simulink model "Traffic_Light_ROS2_NS3_demo"  (R2024b)
settings: Solver=ode3  StartTime=0.0  StopTime=100  FixedStep=0.001  MaxStep=0.05  RelTol=1e-3
model workspace (MAT data in the model file):
  SL_ROS_VariableLengthArrays_MaxSizes.CommonInfo.ArrayTruncateAction = 'EmitWarning'
  SL_ROS_VariableLengthArrays_MaxSizes.MsgTypeMap = containers.Map
  SL_ROS_VariableLengthArrays_MaxSizes.MsgTypeMap.serialization.keys = {'nav_msgs/Path', 'sensor_msgs/Image', 'sensor_msgs/PointCloud2'}
  SL_ROS_VariableLengthArrays_MaxSizes.MsgTypeMap.serialization.values{1}.PropertyName = 'poses'
  SL_ROS_VariableLengthArrays_MaxSizes.MsgTypeMap.serialization.values{1}.DataType = 'geometry_msgs/PoseStamped'
  SL_ROS_VariableLengthArrays_MaxSizes.MsgTypeMap.serialization.values{1}.MaxLength = 1000
  SL_ROS_VariableLengthArrays_MaxSizes.MsgTypeMap.serialization.values{2}(1).PropertyName = 'data'
  SL_ROS_VariableLengthArrays_MaxSizes.MsgTypeMap.serialization.values{2}(1).DataType = 'uint8'
  SL_ROS_VariableLengthArrays_MaxSizes.MsgTypeMap.serialization.values{2}(1).MaxLength = 2000000
  SL_ROS_VariableLengthArrays_MaxSizes.MsgTypeMap.serialization.values{2}(2).PropertyName = 'encoding'
  SL_ROS_VariableLengthArrays_MaxSizes.MsgTypeMap.serialization.values{2}(2).DataType = 'uint8'
  SL_ROS_VariableLengthArrays_MaxSizes.MsgTypeMap.serialization.values{2}(2).MaxLength = 2000000
  SL_ROS_VariableLengthArrays_MaxSizes.MsgTypeMap.serialization.values{3}(1).PropertyName = 'data'
  SL_ROS_VariableLengthArrays_MaxSizes.MsgTypeMap.serialization.values{3}(1).DataType = 'uint8'
  SL_ROS_VariableLengthArrays_MaxSizes.MsgTypeMap.serialization.values{3}(1).MaxLength = 1000000
  SL_ROS_VariableLengthArrays_MaxSizes.MsgTypeMap.serialization.values{3}(2).PropertyName = 'fields'
  SL_ROS_VariableLengthArrays_MaxSizes.MsgTypeMap.serialization.values{3}(2).DataType = 'sensor_msgs/PointField'
  SL_ROS_VariableLengthArrays_MaxSizes.MsgTypeMap.serialization.values{3}(2).MaxLength = 16
  SL_ROS_VariableLengthArrays_MaxSizes.MsgTypeMap.serialization.uniformity = 0
  SL_ROS_VariableLengthArrays_MaxSizes.MsgTypeMap.serialization.keyType = 'char'
  SL_ROS_VariableLengthArrays_MaxSizes.MsgTypeMap.serialization.valueType = 'any'
undefined symbols (not defined in the file or in its folder): brake, gear, hand_brake, manual_gear_shift, reverse, steer, throttle
libraries: ros2lib x5, slpidlib x1, instrumentlib x1
settings Model: PacingRate=0.010000  Creator=iotav  LastModifiedBy=hnh21
settings OptimizationCC: DefaultParameterBehavior=Inlined  EnhancedBackFolding=on  PassReuseOutputArgsAs=Individual arguments  ZeroExternalMemoryAtStartup=off  ZeroInternalMemoryAtStartup=off  MaxStackSize=64  OptimizeBlockOrder=speed  DifferentSizesBufferReuse=on  EfficientTunableParamExpr=on
settings DebuggingCC: ParameterTunabilityLossMsg=error
settings HardwareCC: ProdBitPerLong=64  ProdHWDeviceType=Intel->x86-64 (Linux 64)
settings RTWCC: Description=Embedded Coder  SystemTargetFile=ert.tlc  HardwareBoard=Robot Operating System 2 (ROS 2)  TLCOptions="-aInlineSetEventsForThisBaseRateFcn=TLC_FALSE -aSuppressMultiTaskScheduler=TLC_FALSE  -aRateBasedStepFcn=0"  TemplateMakefile=ert_default_tmf  Toolchain=Colcon Tools  TargetLang=C++
settings CodeAppCC: ForceParamTrailComments=on  IgnoreCustomStorageClasses=off  OperatorAnnotations=on  SimulinkDataObjDesc=on  SFDataObjDesc=on  InsertBlockDesc=on
settings ERTTargetCC: CodeInterfacePackaging=C++ class  RootIOFormat=Structure reference

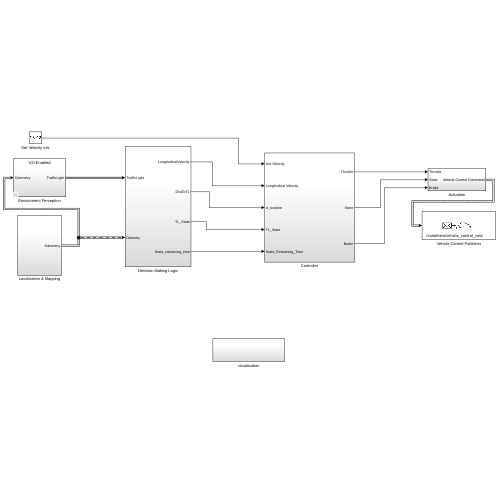
[thumbnail: Simulink's stored preview of the top-level diagram]
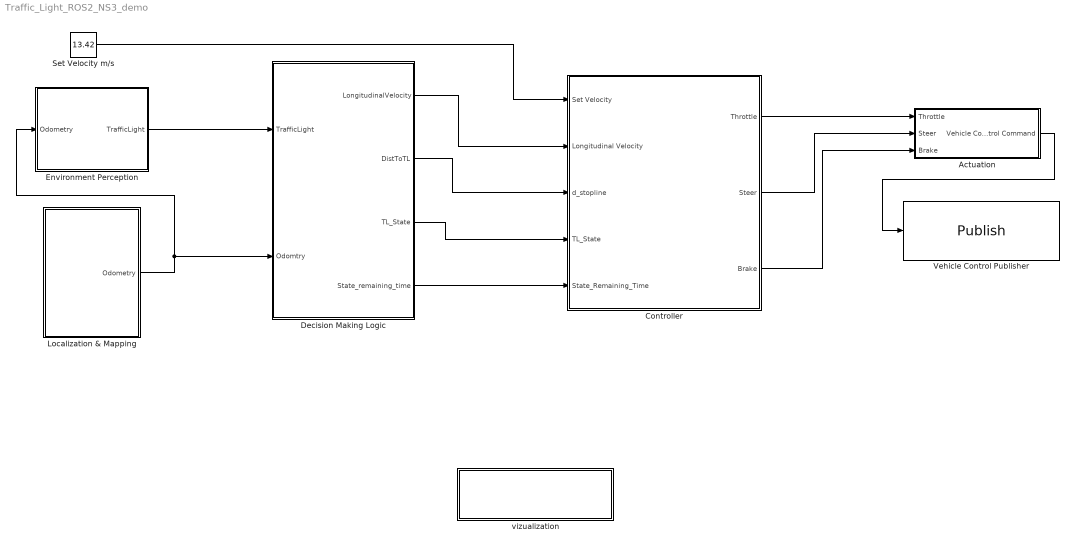
== system Traffic_Light_ROS2_NS3_demo ==
  Actuation : Subsystem
  Controller : Subsystem
  Decision Making Logic : Subsystem
  Environment Perception : Subsystem  Variant=on
  Localization & Mapping : Subsystem
  Set Velocity m/s : Constant  Value=13.42
  Vehicle Control Publisher : ros2lib/Publish  topicSource=Select from ROS network  topic=/carla/hero/vehicle_control_cmd  messageType=carla_msgs/CarlaEgoVehicleControl  QOSHistory=Keep last  QOSDepth=1  QOSReliability=Reliable  QOSDurability=Volatile  QOSDeadline=Inf  QOSLifespan=Inf  QOSLiveliness=Automatic  QOSLeaseDuration=Inf  QOSAvoidROSNamespaceConventions=off
  vizualization : Subsystem
  wires:
  Environment Perception/1(TrafficLight) -> Decision Making Logic/1(TrafficLight)
  Localization & Mapping/1(Odometry) -> Environment Perception/1(Odometry), Decision Making Logic/2(Odomtry)
  Actuation/1(Vehicle Control Command) -> Vehicle Control Publisher/1
  Set Velocity m/s/1 -> Controller/1(Set Velocity)
  Decision Making Logic/1(LongitudinalVelocity) -> Controller/2(Longitudinal Velocity)
  Decision Making Logic/2(DistToTL) -> Controller/3(d_stopline)
  Decision Making Logic/3(TL_State) -> Controller/4(TL_State)
  Controller/1(Throttle) -> Actuation/1(Throttle)
  Controller/2(Steer) -> Actuation/2(Steer)
  Controller/3(Brake) -> Actuation/3(Brake)
  Decision Making Logic/4(State_remaining_time) -> Controller/5(State_Remaining_Time)

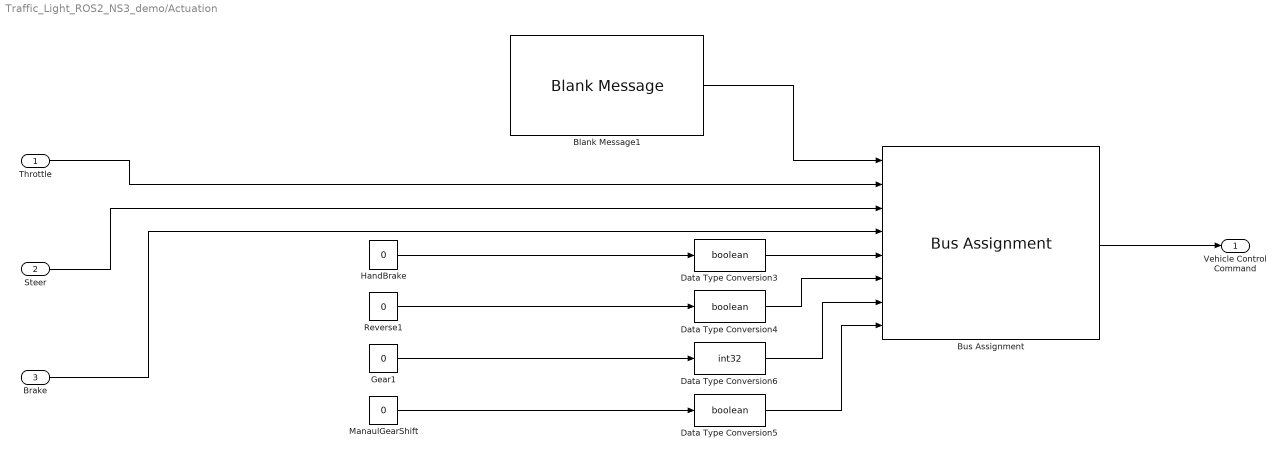
== system Traffic_Light_ROS2_NS3_demo/Actuation ==
  Throttle : Inport
  Steer : Inport  Port=2
  Brake : Inport  Port=3
  Blank Message1 : ros2lib/Blank Message  messageClass=Message  entityType=carla_msgs/CarlaEgoVehicleControl  messageType=carla_msgs/CarlaEgoVehicleControl  SampleTime=inf
  Bus Assignment : BusAssignment  AssignedSignals=throttle,steer,brake,hand_brake,reverse,gear,manual_gear_shift
  Data Type Conversion3 : DataTypeConversion  OutDataTypeStr=boolean  SaturateOnIntegerOverflow=off  RndMeth=Floor
  Data Type Conversion4 : DataTypeConversion  OutDataTypeStr=boolean  SaturateOnIntegerOverflow=off  RndMeth=Floor
  Data Type Conversion5 : DataTypeConversion  OutDataTypeStr=boolean  SaturateOnIntegerOverflow=off  RndMeth=Floor
  Data Type Conversion6 : DataTypeConversion  OutDataTypeStr=int32  SaturateOnIntegerOverflow=off  RndMeth=Floor
  Gear1 : Constant  Value=0  OutDataTypeStr=single
  HandBrake : Constant  Value=0  OutDataTypeStr=single
  ManaulGearShift : Constant  Value=0  OutDataTypeStr=single
  Reverse1 : Constant  Value=0  OutDataTypeStr=single
  Vehicle Control Command : Outport
  wires:
  Data Type Conversion5/1 -> Bus Assignment/8
  Data Type Conversion6/1 -> Bus Assignment/7
  Blank Message1/1 -> Bus Assignment/1
  Data Type Conversion4/1 -> Bus Assignment/6
  Data Type Conversion3/1 -> Bus Assignment/5
  Throttle/1 -> Bus Assignment/2
  Bus Assignment/1 -> Vehicle Control Command/1
  Steer/1 -> Bus Assignment/3
  Brake/1 -> Bus Assignment/4
  HandBrake/1 -> Data Type Conversion3/1
  Reverse1/1 -> Data Type Conversion4/1
  Gear1/1 -> Data Type Conversion6/1
  ManaulGearShift/1 -> Data Type Conversion5/1

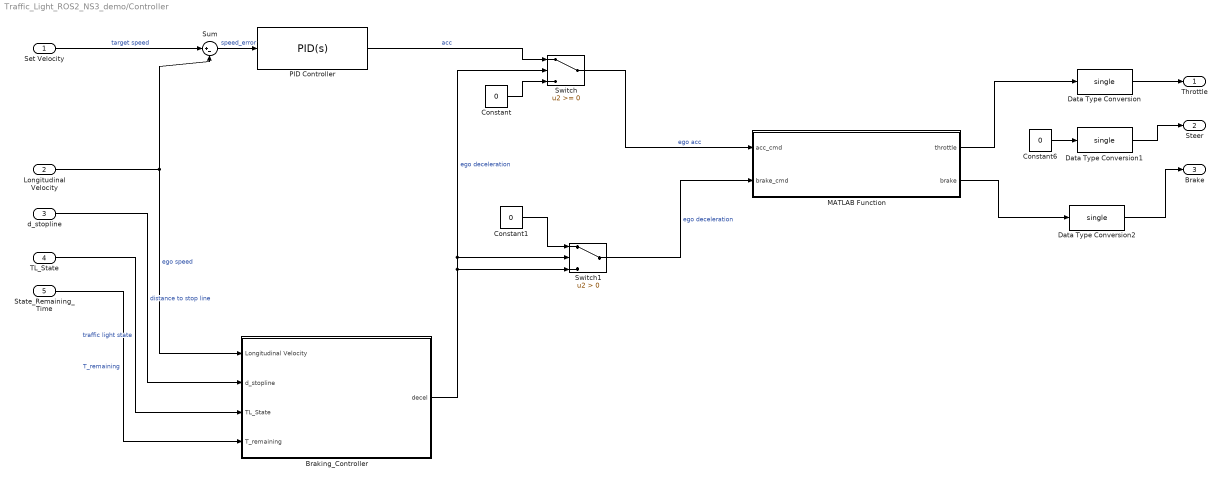
== system Traffic_Light_ROS2_NS3_demo/Controller ==
  Set Velocity : Inport
  Longitudinal Velocity : Inport  Port=2
  d_stopline : Inport  Port=3
  TL_State : Inport  Port=4
  State_Remaining_Time : Inport  Port=5
  Braking_Controller : Subsystem  Variant=on  VariantControl=BRAKING_MODE
  Constant : Constant  Value=0
  Constant1 : Constant  Value=0
  Constant6 : Constant  Value=0
  Data Type Conversion : DataTypeConversion  OutDataTypeStr=single  SaturateOnIntegerOverflow=off  RndMeth=Floor
  Data Type Conversion1 : DataTypeConversion  OutDataTypeStr=single  SaturateOnIntegerOverflow=off  RndMeth=Floor
  Data Type Conversion2 : DataTypeConversion  OutDataTypeStr=single  SaturateOnIntegerOverflow=off  RndMeth=Floor
  MATLAB Function : MATLAB Function  TreatAsAtomicUnit=on
  PID Controller : slpidlib/PID Controller  Controller=PID  Form=Parallel  TimeDomain=Continuous-time  UseExternalTs=off  SampleTime=-1  IntegratorMethod=Forward Euler  FilterMethod=Forward Euler  ControllerParametersSource=internal  P=0.6  I=0.1  UseKiTs=off  D=0  UseExternalDerivativeSource=off  N=100  UseFilter=on  TunerSelectOption=Transfer Function Based (PID Tuner App)  InitialConditionSource=internal  InitialConditionForIntegrator=0  InitialConditionForFilter=0  DifferentiatorICPrevScaledInput=0  ExternalReset=none  TrackingMode=off  Kt=1  LimitOutput=on  SatLimitsSource=internal  UpperSaturationLimit=2  LowerSaturationLimit=-3  LinearizeAsGain=on  AntiWindupMode=none  Kb=1  LimitIntegrator=off  UpperIntegratorSaturationLimit=inf  LowerIntegratorSaturationLimit=-inf  POutMin=[]  POutMax=[]  IOutMin=[]  IOutMax=[]  DOutMin=[]  DOutMax=[]  NOutMin=[]  NOutMax=[]  SumOutMin=[]  SumOutMax=[]  SaturationOutMin=[]  SaturationOutMax=[]  PParamMin=[]  PParamMax=[]  IParamMin=[]  IParamMax=[]  DParamMin=[]  DParamMax=[]  NParamMin=[]  NParamMax=[]  KbParamMin=[]  KbParamMax=[]  KtParamMin=[]  KtParamMax=[]  KbOutMin=[]  KbOutMax=[]  KtOutMin=[]  KtOutMax=[]  IntegratorOutMin=[]  IntegratorOutMax=[]  FilterOutMin=[]  FilterOutMax=[]  SumI1OutMin=[]  SumI1OutMax=[]  SumI2OutMin=[]  SumI2OutMax=[]  SumI3OutMin=[]  SumI3OutMax=[]  SumI4OutMin=[]  SumI4OutMax=[]  SumDOutMin=[]  SumDOutMax=[]  DifferentiatorOutMin=[]  DifferentiatorOutMax=[]  FilterDiffOutCoefMin=[]  FilterDiffOutCoefMax=[]  ReciprocalOutMin=[]  ReciprocalOutMax=[]  SumDenOutMin=[]  SumDenOutMax=[]  SumNumOutMin=[]  SumNumOutMax=[]  DivideOutMin=[]  DivideOutMax=[]  UdiffTsProdOutMin=[]  UdiffTsProdOutMax=[]  NTsProdOutMin=[]  NTsProdOutMax=[]  UintegralTsProdOutMin=[]  UintegralTsProdOutMax=[]  UngainTsProdOutMin=[]  UngainTsProdOutMax=[]  ClampingZeroOutDataTypeStr=Inherit: Inherit via back propagation  ClampingZeroOutMin=[]  ClampingZeroOutMax=[]  FilterDenConstantOutDataTypeStr=Inherit: Inherit via back propagation  FilterDenConstantOutMin=[]  FilterDenConstantOutMax=[]  PCopyOutDataTypeStr=Inherit: Inherit via back propagation  PCopyOutMin=[]  PCopyOutMax=[]  NCopyOutDataTypeStr=Inherit: Inherit via back propagation  NCopyOutMin=[]  NCopyOutMax=[]  IntegratorContinuousStateAttributes=''  IntegratorStateMustResolveToSignalObject=off  IntegratorRTWStateStorageClass=Auto  FilterContinuousStateAttributes=''  FilterStateMustResolveToSignalObject=off  FilterRTWStateStorageClass=Auto  ParallelPVariant=InternalParameters  IdealPVariant=Disabled  IVariant=InternalParameters  DVariant=InternalParameters  IntegratorVariant=Continuous  SatVariant=Enabled  AWVariant=Passthrough  PCopyVariant=Disabled  TRVariant=Disabled  FdbkBlocksVariant=Forward  IdealPFdbkVariant=Disabled  SatFdbkVariant=Disabled  DerivativeFilterVariant=ContFilter  NVariant=InternalParameters  NCopyVariant=Disabled  FilterICVariant=InternalICsFilter  IntegratorICVariant=InternalICs  ExternalResetVariant=Disabled  TRSumVariant=Passthrough  SumFdbkVariant=Disabled  SumVariant=Sum_PID  TsampFilterVariant=InternalTs  TsampNgainVariant=Passthrough  TsampIntegralVariant=Disabled_SignalSpec  ExternalSaturationOutDataTypeStr=Inherit: Same as second input  DerivativeSourceVariant=ErrorSignal  PreIntVariant=InternalPreInt
  Sum : Sum  Inputs=|+-
  Switch : Switch  SaturateOnIntegerOverflow=off  InputSameDT=off
  Switch1 : Switch  Criteria=u2 > Threshold  SaturateOnIntegerOverflow=off  InputSameDT=off
  Throttle : Outport
  Steer : Outport  Port=2
  Brake : Outport  Port=3
  wires:
  Constant6/1 -> Data Type Conversion1/1
  d_stopline/1 -> Braking_Controller/2(d_stopline)  "distance to stop line"
  MATLAB Function/1(throttle) -> Data Type Conversion/1
  Set Velocity/1 -> Sum/1  "target speed"
  Data Type Conversion2/1 -> Brake/1
  Sum/1 -> PID Controller/1  "speed_error"
  TL_State/1 -> Braking_Controller/3(TL_State)  "traffic light state"
  MATLAB Function/2(brake) -> Data Type Conversion2/1
  Data Type Conversion/1 -> Throttle/1
  Braking_Controller/1(decel) -> Switch1/3, Switch/2, Switch1/2  "ego deceleration"
  Data Type Conversion1/1 -> Steer/1
  Longitudinal Velocity/1 -> Braking_Controller/1(Longitudinal Velocity), Sum/2  "ego speed"
  PID Controller/1 -> Switch/1  "acc"
  Switch/1 -> MATLAB Function/1(acc_cmd)  "ego acc"
  Constant/1 -> Switch/3
  State_Remaining_Time/1 -> Braking_Controller/4(T_remaining)  "T_remaining"
  Switch1/1 -> MATLAB Function/2(brake_cmd)  "ego deceleration"
  Constant1/1 -> Switch1/1

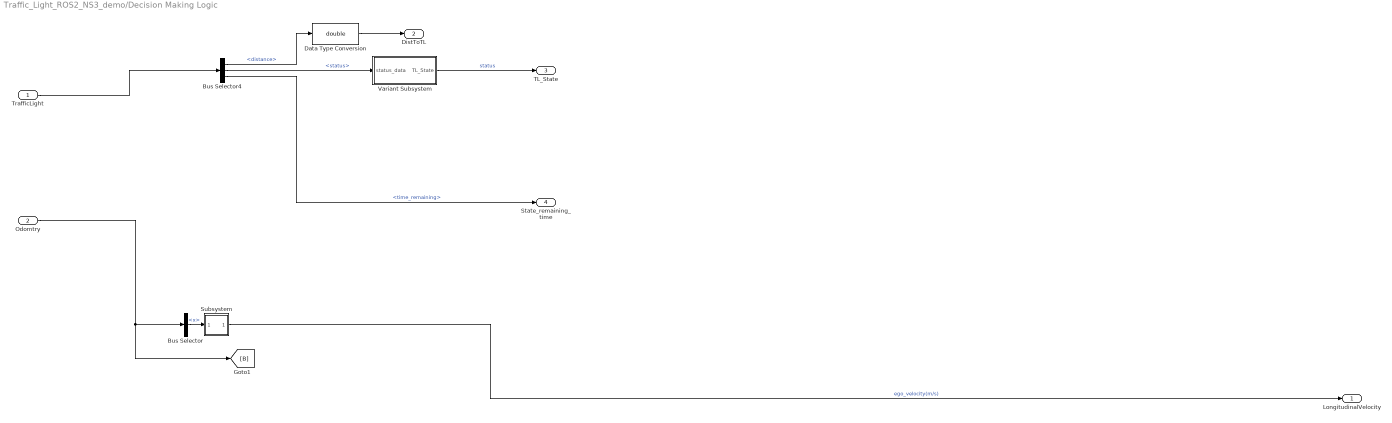
== system Traffic_Light_ROS2_NS3_demo/Decision Making Logic ==
  TrafficLight : Inport
  Odomtry : Inport  Port=2
  Bus Selector : BusSelector  OutputSignals=twist.twist.linear.x
  Bus Selector4 : BusSelector  OutputSignals=distance,status,time_remaining
  Data Type Conversion : DataTypeConversion  OutDataTypeStr=double  SaturateOnIntegerOverflow=off  RndMeth=Floor
  Subsystem : Subsystem
  Variant Subsystem : Subsystem  Variant=on
  LongitudinalVelocity : Outport
  DistToTL : Outport  Port=2
  TL_State : Outport  Port=3
  State_remaining_time : Outport  Port=4
  wires:
  Subsystem/1(Out1) -> LongitudinalVelocity/1  "ego_velocity(m/s)"
  Odomtry/1 -> [B], Bus Selector/1
  Bus Selector/1 -> Subsystem/1(In1)  "<x>"
  TrafficLight/1 -> Bus Selector4/1
  Bus Selector4/2 -> Variant Subsystem/1(status_data)  "<status>"
  Bus Selector4/1 -> Data Type Conversion/1  "<distance>"
  Bus Selector4/3 -> State_remaining_time/1  "<time_remaining>"
  Variant Subsystem/1(TL_State) -> TL_State/1  "status"
  Data Type Conversion/1 -> DistToTL/1

== system Traffic_Light_ROS2_NS3_demo/Environment Perception ==
  note: 1) Add Subsystem or Model blocks as valid variant choices.
      | 2) You cannot connect blocks at this level. At simulation, connectivity is automatically
      | determined, based on the active variant and port name matching.
  Odometry : Inport
  Perception-Based : Subsystem  VariantControl=BRAKING_MODE ==1
  V2I-Enabled : Subsystem  TreatAsAtomicUnit=on  VariantControl=BRAKING_MODE ==2
  TrafficLight : Outport

== system Traffic_Light_ROS2_NS3_demo/Localization & Mapping ==
  Subscribe : ros2lib/Subscribe  topicSource=Select from ROS network  topic=/carla/hero/odometry  messageType=nav_msgs/Odometry  sampleTime=-1  QOSHistory=Keep last  QOSDepth=1  QOSReliability=Reliable  QOSDurability=Volatile  QOSDeadline=Inf  QOSLifespan=Inf  QOSLiveliness=Automatic  QOSLeaseDuration=Inf  QOSAvoidROSNamespaceConventions=off
  Terminator3 : Terminator
  Odometry : Outport
  wires:
  Subscribe/1 -> Terminator3/1
  Subscribe/2 -> Odometry/1

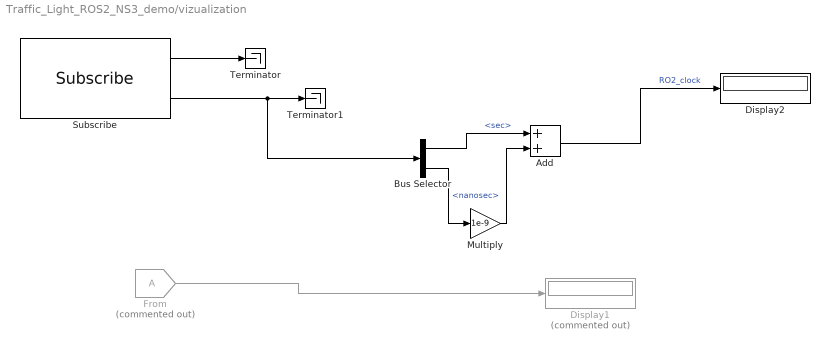
== system Traffic_Light_ROS2_NS3_demo/vizualization ==
  Add : Sum
  Bus Selector : BusSelector  OutputSignals=clock.sec,clock.nanosec
  Display1 : Display  Commented=on
  Display2 : Display
  From : From  Commented=on  TagVisibility=global
  Multiply : Gain  Gain=1e-9
  Subscribe : ros2lib/Subscribe  topicSource=Select from ROS network  topic=/clock  messageType=rosgraph_msgs/Clock  sampleTime=-1  QOSHistory=Keep last  QOSDepth=1  QOSReliability=Reliable  QOSDurability=Volatile  QOSDeadline=Inf  QOSLifespan=Inf  QOSLiveliness=Automatic  QOSLeaseDuration=Inf  QOSAvoidROSNamespaceConventions=off
  Terminator : Terminator
  Terminator1 : Terminator
  wires:
  Subscribe/2 -> Bus Selector/1, Terminator1/1
  Subscribe/1 -> Terminator/1
  From/1 -> Display1/1
  Bus Selector/1 -> Add/1  "<sec>"
  Bus Selector/2 -> Multiply/1  "<nanosec>"
  Add/1 -> Display2/1  "RO2_clock"
  Multiply/1 -> Add/2

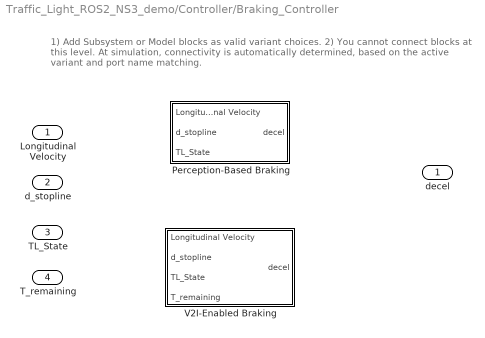
== system Traffic_Light_ROS2_NS3_demo/Controller/Braking_Controller ==
  note: 1) Add Subsystem or Model blocks as valid variant choices.
      | 2) You cannot connect blocks at this level. At simulation, connectivity is automatically
      | determined, based on the active variant and port name matching.
  Longitudinal Velocity : Inport
  d_stopline : Inport  Port=2
  TL_State : Inport  Port=3
  T_remaining : Inport  Port=4
  Perception-Based Braking : Subsystem  VariantControl=BRAKING_MODE == 1
  V2I-Enabled Braking : Subsystem  VariantControl=BRAKING_MODE == 2
  decel : Outport

== system Traffic_Light_ROS2_NS3_demo/Decision Making Logic/Subsystem ==
  In1 : Inport
  Out1 : Outport
  wires:
  In1/1 -> Out1/1

== system Traffic_Light_ROS2_NS3_demo/Decision Making Logic/Variant Subsystem ==
  note: 1) Add Subsystem or Model blocks as valid variant choices.
      | 2) You cannot connect blocks at this level. At simulation, connectivity is automatically
      | determined, based on the active variant and port name matching.
  status_data : Inport
  Perception-Based : Subsystem  VariantControl=BRAKING_MODE ==1
  V2I-Enabled : Subsystem  VariantControl=BRAKING_MODE ==2
  TL_State : Outport

== system Traffic_Light_ROS2_NS3_demo/Environment Perception/Perception-Based ==
  Bus Selector : BusSelector  OutputSignals=signal1,signal2
  Subscribe : ros2lib/Subscribe  topicSource=Select from ROS network  topic=/carla/hero/traffic_light_in_front  messageType=carla_msgs/TrafficLightInfo  sampleTime=-1  QOSHistory=Keep last  QOSDepth=1  QOSReliability=Reliable  QOSDurability=Volatile  QOSDeadline=Inf  QOSLifespan=Inf  QOSLiveliness=Automatic  QOSLeaseDuration=Inf  QOSAvoidROSNamespaceConventions=off
  Terminator1 : Terminator
  TrafficLight : Outport
  wires:
  Subscribe/1 -> Terminator1/1
  Subscribe/2 -> TrafficLight/1, Bus Selector/1

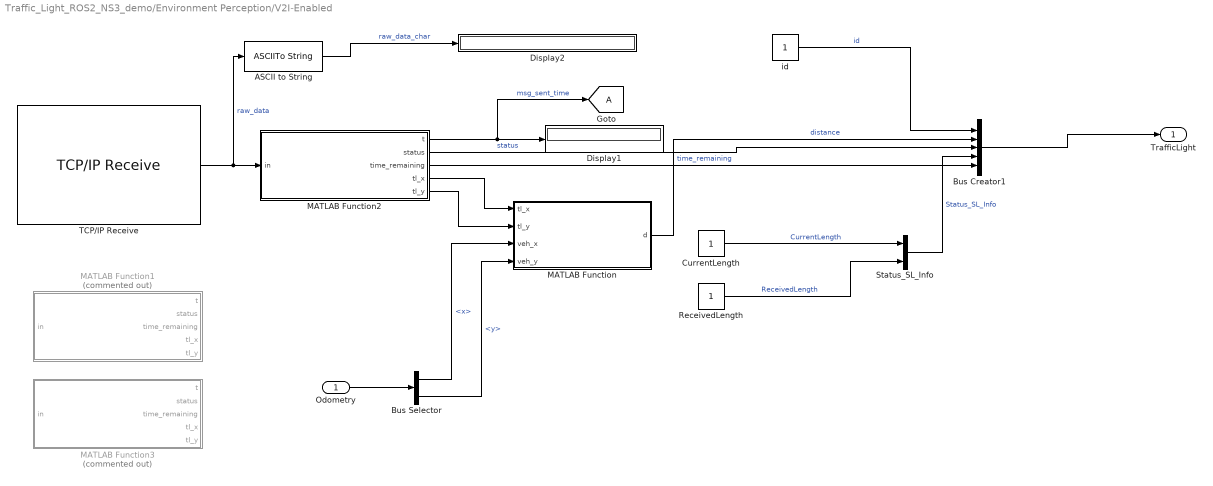
== system Traffic_Light_ROS2_NS3_demo/Environment Perception/V2I-Enabled ==
  Odometry : Inport
  ASCII to String : ASCIIToString
  Bus Creator1 : BusCreator  Inputs=5
  Bus Selector : BusSelector  OutputSignals=pose.pose.position.x,pose.pose.position.y
  CurrentLength : Constant
  Display1 : Display
  Display2 : Display
  Goto : Goto  TagVisibility=global
  MATLAB Function : MATLAB Function  TreatAsAtomicUnit=on
  MATLAB Function1 : MATLAB Function  Commented=on  TreatAsAtomicUnit=on
  MATLAB Function2 : MATLAB Function  TreatAsAtomicUnit=on
  MATLAB Function3 : MATLAB Function  Commented=on  TreatAsAtomicUnit=on
  ReceivedLength : Constant
  Status_SL_Info : BusCreator  Inputs=2
  TCP/IP Receive : instrumentlib/TCP//IP Receive  Host=127.0.0.1  Port=9000  DataSize=38  DataType=uint8  ASCIIFormatting=%f  Terminator=LF  CustomTerminator=10  ByteOrder=big-endian  EnableBlockingMode=on  Timeout=0.5  SampleTime=0.001  SimulateUsing=Interpreted execution
  id : Constant
  TrafficLight : Outport
  wires:
  CurrentLength/1 -> Status_SL_Info/1  "CurrentLength"
  ReceivedLength/1 -> Status_SL_Info/2  "ReceivedLength"
  id/1 -> Bus Creator1/1  "id"
  MATLAB Function/1(d) -> Bus Creator1/2  "distance"
  MATLAB Function2/2(status) -> Bus Creator1/3  "status"
  Status_SL_Info/1 -> Bus Creator1/4  "Status_SL_Info"
  MATLAB Function2/3(time_remaining) -> Bus Creator1/5  "time_remaining"
  Bus Creator1/1 -> TrafficLight/1
  TCP/IP Receive/1 -> ASCII to String/1, MATLAB Function2/1(in)  "raw_data"
  Odometry/1 -> Bus Selector/1
  Bus Selector/2 -> MATLAB Function/4(veh_y)  "<y>"
  Bus Selector/1 -> MATLAB Function/3(veh_x)  "<x>"
  MATLAB Function2/4(tl_x) -> MATLAB Function/1(tl_x)
  MATLAB Function2/5(tl_y) -> MATLAB Function/2(tl_y)
  MATLAB Function2/1(t) -> Goto/1, Display1/1  "msg_sent_time"
  ASCII to String/1 -> Display2/1  "raw_data_char"

== system Traffic_Light_ROS2_NS3_demo/Controller/Braking_Controller/Perception-Based Braking ==
  Longitudinal Velocity : Inport
  d_stopline : Inport  Port=2
  TL_State : Inport  Port=3
  Brake Distance Calculation : Subsystem
  BrakingLogic : Subsystem
  decel : Outport
  wires:
  Brake Distance Calculation/1(d_comfort) -> BrakingLogic/2(d_comfort)  "distance comfort"
  TL_State/1 -> BrakingLogic/4(TL_State)
  Longitudinal Velocity/1 -> Brake Distance Calculation/1(Longitudinal speed), BrakingLogic/1(longVelocity)
  d_stopline/1 -> BrakingLogic/3(d_stopline)
  BrakingLogic/1(decel) -> decel/1

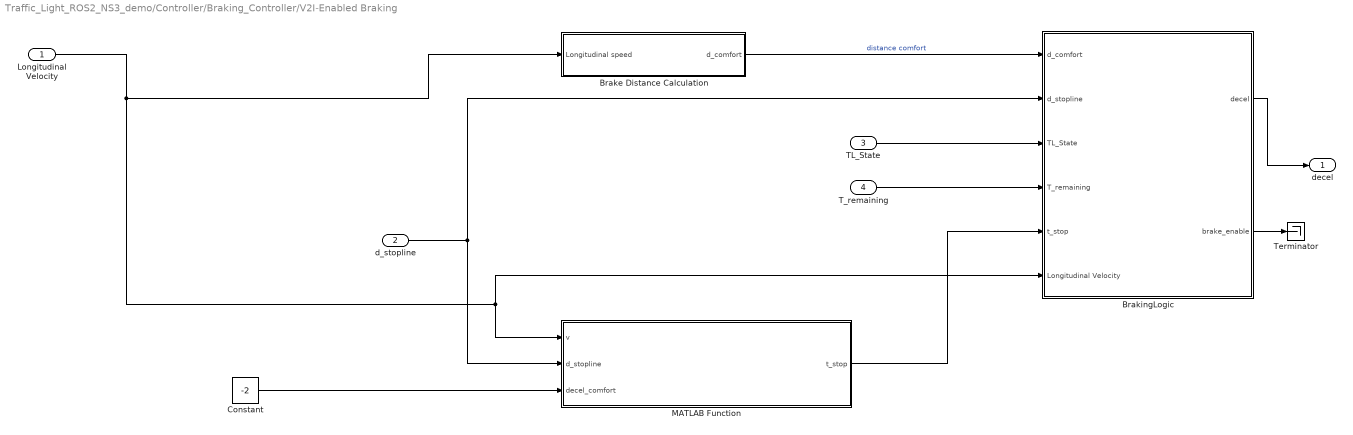
== system Traffic_Light_ROS2_NS3_demo/Controller/Braking_Controller/V2I-Enabled Braking ==
  Longitudinal Velocity : Inport
  d_stopline : Inport  Port=2
  TL_State : Inport  Port=3
  T_remaining : Inport  Port=4
  Brake Distance Calculation : Subsystem
  BrakingLogic : Subsystem
  Constant : Constant  Value=-2
  MATLAB Function : MATLAB Function  TreatAsAtomicUnit=on
  Terminator : Terminator
  decel : Outport
  wires:
  T_remaining/1 -> BrakingLogic/4(T_remaining)
  Brake Distance Calculation/1(d_comfort) -> BrakingLogic/1(d_comfort)  "distance comfort"
  TL_State/1 -> BrakingLogic/3(TL_State)
  d_stopline/1 -> MATLAB Function/2(d_stopline), BrakingLogic/2(d_stopline)
  Longitudinal Velocity/1 -> MATLAB Function/1(v), BrakingLogic/6(Longitudinal Velocity), Brake Distance Calculation/1(Longitudinal speed)
  BrakingLogic/1(decel) -> decel/1
  BrakingLogic/2(brake_enable) -> Terminator/1
  Constant/1 -> MATLAB Function/3(decel_comfort)
  MATLAB Function/1(t_stop) -> BrakingLogic/5(t_stop)

== system Traffic_Light_ROS2_NS3_demo/Decision Making Logic/Variant Subsystem/Perception-Based ==
  status_data : Inport
  MATLAB Function2 : MATLAB Function  TreatAsAtomicUnit=on
  TL_State : Outport
  wires:
  status_data/1 -> MATLAB Function2/1(status_data)
  MATLAB Function2/1(traffic_status_code) -> TL_State/1  "status"

== system Traffic_Light_ROS2_NS3_demo/Decision Making Logic/Variant Subsystem/V2I-Enabled ==
  status_data : Inport
  TL_State : Outport
  wires:
  status_data/1 -> TL_State/1

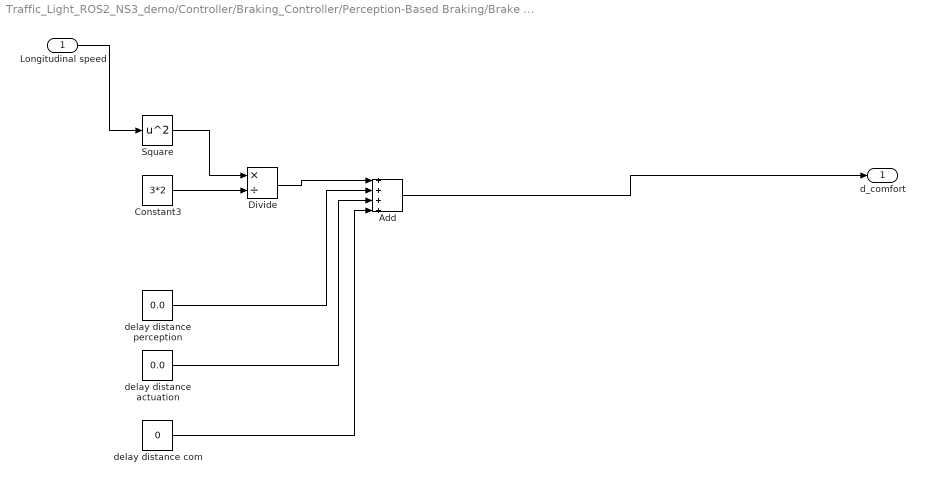
== system Traffic_Light_ROS2_NS3_demo/Controller/Braking_Controller/Perception-Based Braking/Brake Distance Calculation ==
  Longitudinal speed : Inport
  Add : Sum  Inputs=++++
  Constant3 : Constant  Value=3*2
  Divide : Product  Inputs=*/
  Square : Math  Operator=square
  delay distance actuation : Constant  Value=0.0
  delay distance com : Constant  Value=0
  delay distance perception : Constant  Value=0.0
  d_comfort : Outport
  wires:
  Divide/1 -> Add/1
  Constant3/1 -> Divide/2
  delay distance perception/1 -> Add/2
  delay distance com/1 -> Add/4
  Add/1 -> d_comfort/1
  delay distance actuation/1 -> Add/3
  Square/1 -> Divide/1
  Longitudinal speed/1 -> Square/1

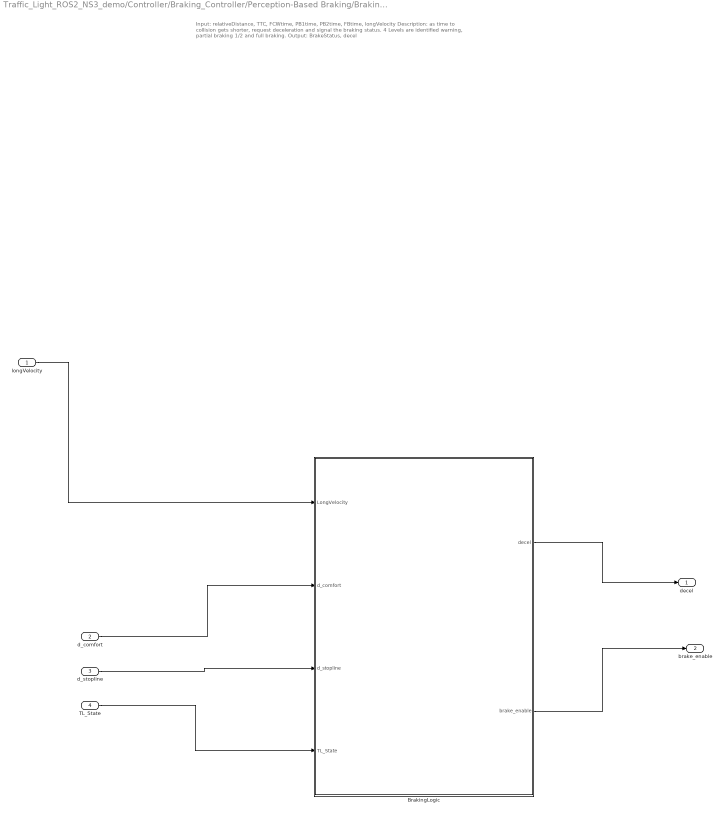
== system Traffic_Light_ROS2_NS3_demo/Controller/Braking_Controller/Perception-Based Braking/BrakingLogic ==
  note: Input: relativeDistance, TTC, FCWtime, PB1time, PB2time, FBtime, longVelocity
      | Description: as time to collision gets shorter, request deceleration and signal the braking status. 4 Levels are identified warning, partial braking 1/2 and full braking.
      | Output: BrakeStatus, decel
  longVelocity : Inport
  d_comfort : Inport  Port=2
  d_stopline : Inport  Port=3
  TL_State : Inport  Port=4
  BrakingLogic : Stateflow chart  TreatAsAtomicUnit=on
  decel : Outport
  brake_enable : Outport  Port=2
  wires:
  longVelocity/1 -> BrakingLogic/1(LongVelocity)
  d_stopline/1 -> BrakingLogic/3(d_stopline)
  TL_State/1 -> BrakingLogic/4(TL_State)
  BrakingLogic/1(decel) -> decel/1
  BrakingLogic/2(brake_enable) -> brake_enable/1
  d_comfort/1 -> BrakingLogic/2(d_comfort)

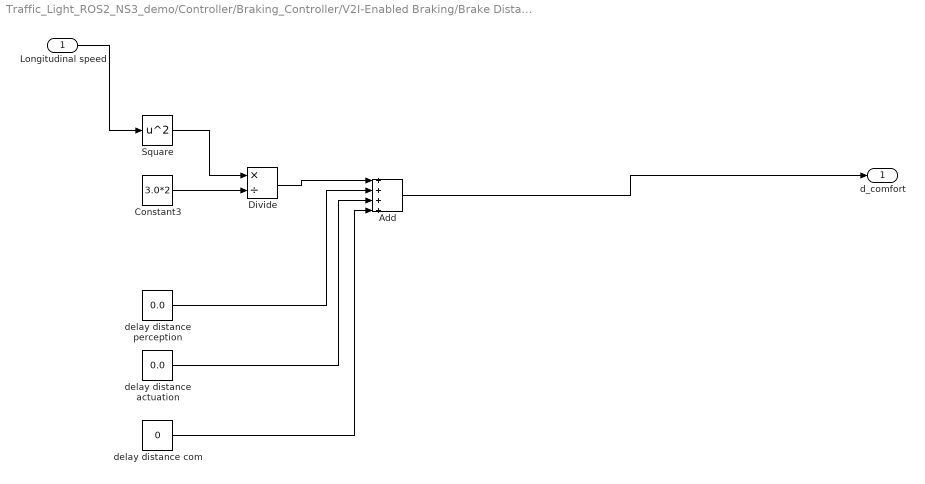
== system Traffic_Light_ROS2_NS3_demo/Controller/Braking_Controller/V2I-Enabled Braking/Brake Distance Calculation ==
  Longitudinal speed : Inport
  Add : Sum  Inputs=++++
  Constant3 : Constant  Value=3.0*2
  Divide : Product  Inputs=*/
  Square : Math  Operator=square
  delay distance actuation : Constant  Value=0.0
  delay distance com : Constant  Value=0
  delay distance perception : Constant  Value=0.0
  d_comfort : Outport
  wires:
  Divide/1 -> Add/1
  Constant3/1 -> Divide/2
  delay distance perception/1 -> Add/2
  delay distance com/1 -> Add/4
  Add/1 -> d_comfort/1
  delay distance actuation/1 -> Add/3
  Square/1 -> Divide/1
  Longitudinal speed/1 -> Square/1

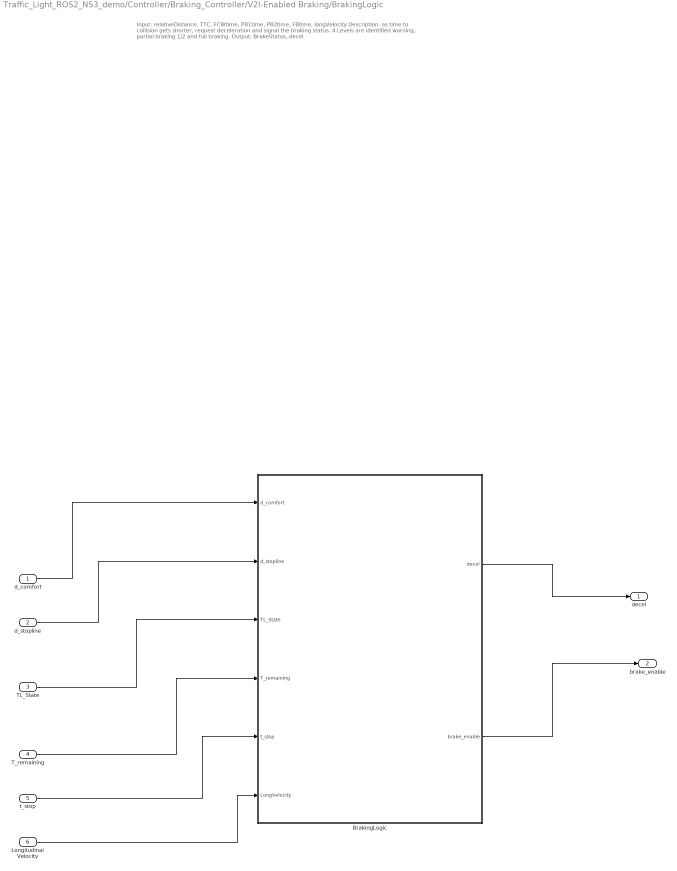
== system Traffic_Light_ROS2_NS3_demo/Controller/Braking_Controller/V2I-Enabled Braking/BrakingLogic ==
  note: Input: relativeDistance, TTC, FCWtime, PB1time, PB2time, FBtime, longVelocity
      | Description: as time to collision gets shorter, request deceleration and signal the braking status. 4 Levels are identified warning, partial braking 1/2 and full braking.
      | Output: BrakeStatus, decel
  d_comfort : Inport
  d_stopline : Inport  Port=2
  TL_State : Inport  Port=3
  T_remaining : Inport  Port=4
  t_stop : Inport  Port=5
  Longitudinal Velocity : Inport  Port=6
  BrakingLogic : Stateflow chart  TreatAsAtomicUnit=on
  decel : Outport
  brake_enable : Outport  Port=2
  wires:
  d_stopline/1 -> BrakingLogic/2(d_stopline)
  TL_State/1 -> BrakingLogic/3(TL_State)
  BrakingLogic/1(decel) -> decel/1
  BrakingLogic/2(brake_enable) -> brake_enable/1
  d_comfort/1 -> BrakingLogic/1(d_comfort)
  T_remaining/1 -> BrakingLogic/4(T_remaining)
  t_stop/1 -> BrakingLogic/5(t_stop)
  Longitudinal Velocity/1 -> BrakingLogic/6(LongVelocity)

== matlab function Traffic_Light_ROS2_NS3_demo/Environment Perception/V2I-Enabled/MATLAB Function2 ==
  data: in input; t output; status output; time_remaining output; tl_x output; tl_y output
function [t, status, time_remaining, tl_x, tl_y] = parseMsg(in)
%#codegen

% Convert byte array to string
line = char(in(:)');  % Turn uint8 to string

% Default values
t = 0.0;
status = 0;
time_remaining = 0.0;
tl_x = 0.0;
tl_y = 0.0;

% Remove newline character
line = strtrim(line);

% Parse if it's well-formed
tokens = sscanf(line, '%f,%d,%f,%f,%f');
if numel(tokens) >= 5
    t = tokens(1);
    status = tokens(2);
    time_remaining = tokens(3);
    tl_x = tokens(4);
    tl_y = tokens(5);
end

== stateflow chart Traffic_Light_ROS2_NS3_demo/Controller/Braking_Controller/Perception-Based Braking/BrakingLogic/BrakingLogic ==
  state Driving
    entry: brake_enable = 0; decel = 0;
  state Braking
    entry: brake_enable = 1;
    during: decel = -min(9.8, LongVelocity^2 / (4* (d_stopline + 2.0)));
  state Stopped
    entry: brake_enable =1; decel = -0.1;
  (default) -> Driving
  Stopped -> Driving : [TL_State ==1]
  Driving -> Braking : [((TL_State == 3) || (TL_State == 2)) && (d_stopline <= d_comfort) && (d_stopline >0.0)]
  Braking -> Stopped : [(d_stopline <= 2.0) && (LongVelocity <=1.0)]
  data: LongVelocity input; d_comfort input; d_stopline input; TL_State input; decel output; brake_enable output double

== matlab function Traffic_Light_ROS2_NS3_demo/Decision Making Logic/Variant Subsystem/Perception-Based/MATLAB Function2 ==
  data: status_data input; traffic_status_code output
function traffic_status_code = decode_traffic_status(status_data)
    % Ensure status_data is treated as a row vector character array
    status_str = char(status_data(:)'); % Convert to row vector

    % Remove null characters (zeros) and trim spaces
    status_str = status_str(status_str ~= 0);
    status_str = strtrim(status_str);

    % Convert to string for compatibility
    status_str = string(status_str); 

    % Assign integer values to traffic statuses
    if contains(status_str, "Green", 'IgnoreCase', true)
        traffic_status_code = double(1); % Green
    elseif contains(status_str, "Yellow", 'IgnoreCase', true)
        traffic_status_code = double(2); % Yellow
    elseif contains(status_str, "Red", 'IgnoreCase', true)
        traffic_status_code = double(3); % Red
    else
        traffic_status_code = double(0); % Unknown
    end
end

== matlab function Traffic_Light_ROS2_NS3_demo/Controller/MATLAB Function ==
  data: acc_cmd input; throttle output; brake output; brake_cmd input
function [throttle, brake] = convertAccelerationToThrottleBrake(acc_cmd, brake_cmd)
    % Define acceleration and deceleration limits based on vehicle dynamics
    max_acceleration = 2.0;   % Maximum acceleration (m/s²)
    max_deceleration = 3.0;   % Maximum ACC deceleration (m/s²)
    max_emergency_braking = 9.8; % Max deceleration for traffic light stop (m/s²)
    
    % Initialize outputs
    throttle = 0.0;
    brake = 0.0;

    % PRIORITY: Traffic Light Braking Logic
    if brake_cmd < 0  % Negative means braking is required
        brake_force = min(abs(brake_cmd) / max_emergency_braking, 1.0);
        throttle = 0;  % Ensure throttle is OFF
        brake = brake_force;  % Apply required braking
        
    % ACC Control (Only if no Traffic Light Braking)
    elseif acc_cmd >= 0  % Positive acceleration (Throttle)
        throttle_force = min(acc_cmd / max_acceleration, 1.0);
        throttle = throttle_force;
        brake = 0;  % Ensure brake is OFF
        
    elseif acc_cmd < 0  % Negative acceleration (ACC Braking)
        brake_force = min(abs(acc_cmd) / max_deceleration, 1.0);
        throttle = 0;  % Ensure throttle is OFF
        brake = brake_force;  % Apply ACC braking
    end

end

== matlab function Traffic_Light_ROS2_NS3_demo/Environment Perception/V2I-Enabled/MATLAB Function ==
  data: tl_x input; d output; tl_y input; veh_x input; veh_y input
function d = computeDistance(tl_x, tl_y, veh_x, veh_y)
%#codegen

% Compute 2D Euclidean distance between vehicle and traffic light
dx = veh_x - tl_x;
dy = veh_y - tl_y;

d = sqrt(dx^2 + dy^2)-27.0;

== matlab function Traffic_Light_ROS2_NS3_demo/Environment Perception/V2I-Enabled/MATLAB Function1 ==
  data: in input; t output; status output; time_remaining output; tl_x output; tl_y output
function [t, status, time_remaining, tl_x, tl_y] = parseMsg(in)
%#codegen

% Define max buffer size
MAX_LEN = 256;

% Persistent buffer and index
persistent buffer idx

if isempty(buffer)
    buffer = zeros(1, MAX_LEN, 'uint8');  % uint8 buffer
    idx = 0;
end

% Initialize outputs
t = 0.0;
status = 0;
time_remaining = 0.0;
tl_x = 0.0;
tl_y = 0.0;

% Process input
for i = 1:length(in)
    b = uint8(in(i));

    if idx < MAX_LEN
        idx = idx + 1;
        buffer(idx) = b;
    end

    if b == 10  % newline
        line = char(buffer(1:idx-1));  % remove newline
        tokens = sscanf(line, '%f,%d,%f,%f,%f');  % read first 5 fields
        if numel(tokens) >= 5
            t = tokens(1);
            status = tokens(2);
            time_remaining = tokens(3);
            tl_x = tokens(4);
            tl_y = tokens(5);
        end
        idx = 0;  % reset buffer
    end
end

== matlab function Traffic_Light_ROS2_NS3_demo/Controller/Braking_Controller/V2I-Enabled Braking/MATLAB Function ==
  data: v input; d_stopline input; t_stop output; decel_comfort input
function t_stop = calculate_t_stop(v, d_stopline, decel_comfort)
    % calculate_t_stop: Computes the time to stop (t_stop) based on vehicle speed,
    % distance to stop line, and comfortable deceleration.
    %
    % Inputs:
    %   v - Vehicle speed (m/s)
    %   d_stopline - Distance to stop line (meters)
    %   decel_comfort - Comfortable deceleration rate (m/s^2, negative value, e.g., -2.0)
    %
    % Output:
    %   t_stop - Time to stop (seconds), or NaN if calculation is invalid
    %
    % Notes:
    %   - Assumes constant deceleration at decel_comfort until stop line is reached.
    %   - Uses the positive root of the quadratic equation.

    % Ensure inputs are valid
    % if nargin < 3 || isempty(v) || isempty(d_stopline) || isempty(decel_comfort)
    %     error('All inputs (v, d_stopline, decel_comfort) must be provided.');
    % end
    % if v < 0.5 || d_stopline < 0
    %     error('Speed (v) and distance (d_stopline) must be non-negative.');
    % end
    % if decel_comfort >= 0
    %     error('decel_comfort must be negative (e.g., -2.0 m/s^2).');
    % end

    % Absolute value of deceleration for calculation
    decel_abs = abs(decel_comfort);

    % Calculate the discriminant
    discriminant = v^2 - 2 * decel_abs * d_stopline;

    % Check if the vehicle can stop within d_stopline
    if discriminant < 0
        warning('Discriminant is negative: Vehicle cannot stop within d_stopline with decel_comfort. Returning NaN.');
        t_stop = NaN;
        return;
    end

    % Calculate t_stop using the positive root
    t_stop = (v + sqrt(discriminant)) / decel_abs;

    % Ensure t_stop is positive
    if t_stop <= 0
        warning('Calculated t_stop is non-positive. Returning NaN.');
        t_stop = NaN;
    end
end

== matlab function Traffic_Light_ROS2_NS3_demo/Environment Perception/V2I-Enabled/MATLAB Function3 ==
  data: in input; t output; status output; time_remaining output; tl_x output; tl_y output
function [t, status, time_remaining, tl_x, tl_y] = parseMsg(in)
%#codegen

MAX_LEN = 256;

persistent buffer idx
if isempty(buffer)
    buffer = zeros(1, MAX_LEN, 'uint8');
    idx = 0;
end

% Initialize outputs
t = 0.0;
status = 0;
time_remaining = 0.0;
tl_x = 0.0;
tl_y = 0.0;

% Declare variable-size for codegen
coder.varsize('line', [1, MAX_LEN], [0 1]);

for i = 1:length(in)
    b = uint8(in(i));

    if idx < MAX_LEN
        idx = idx + 1;
        buffer(idx) = b;
    end

    if b == 10  % newline detected
        newline_idx = idx;
        if newline_idx > 1
            line = char(buffer(1:newline_idx-1));
            tokens = sscanf(line, '%f,%d,%f,%f,%f');
            if numel(tokens) >= 5
                t = tokens(1);
                status = tokens(2);
                time_remaining = tokens(3);
                tl_x = tokens(4);
                tl_y = tokens(5);
            end
        end
        idx = 0;  % reset buffer
    end
end

== stateflow chart Traffic_Light_ROS2_NS3_demo/Controller/Braking_Controller/V2I-Enabled Braking/BrakingLogic/BrakingLogic ==
  state Driving
    entry: brake_enable = 0; decel = 0;
  state Braking
    entry: brake_enable = 1;
    %during: decel = -9.8 *((d_comfort - d_stopline)^2/d_comfort^2)
    during: decel = -min(9.8, LongVelocity^2 / (4* (d_stopline + 2.00)));
  state Stopped
    entry: brake_enable =1; decel = -0.1;
  (default) -> Driving
  Stopped -> Driving : [TL_State ==1]
  Driving -> Braking : [(TL_State == 1 && T_remaining <= t_stop && d_stopline <= d_comfort) || (((TL_State ==2) || (TL_State == 3)) && d_stopline <= d_comfort && d_stopline >0)]
  Braking -> Stopped : [(d_stopline <= 2.0) && (LongVelocity <=1.0)]
  data: d_comfort input; d_stopline input; TL_State input; decel output; brake_enable output double; T_remaining input; t_stop input; LongVelocity input
